simulink model "LATC_Test_Calc5000000"  (R2020b)
settings: Solver=FixedStepDiscrete  StartTime=4067.8601  StopTime=4107.8798  FixedStep=0.02  RelTol=1e-3
libraries: simulink x8
(part 2 of 2)

== matlab function LATC_Test_Calc5000000/MATLAB Function ==
  data: input input; y output; reset input; Tau input; b input; Ts input
function y = LatCtrlLeadFilter(input, reset, Tau, b, Ts)
%#codegen
%Description: Discrete implementation of the continious lead filter 
%G_lead_continious = (1+s*Tau)/(1+s*Tau) using Tustin transformation 
%(also known as bilinear transformation), hence s=2*(z-1)/(Ts*(z+1));

%--------------Inputs----------------------------------------------
%input                  input to lead filter
%reset                  Boolean indicating whether to reset the system
%Tau                    lead filter parameter, see Description section
%b                      Lead filter parameter, see Description section
% b=cot(Ts*wc/2)  双移线性变换 wc为截至频率
%Ts                     Sample time
%-------------------------------------------------------------------

%--------------Outputs----------------------------------------------
%y                     the output from the lead filter
%-------------------------------------------------------------------
persistent input_prev;
persistent output_prev;


if isempty(input_prev)
    input_prev = single(0);
end

if isempty(output_prev)
    output_prev = single(0);
end

if reset
    y = input;
else
    d1 = (b*Ts+2*Tau*b)/(b*Ts+2*Tau);
    d2 = (b*Ts-2*Tau*b)/(b*Ts+2*Tau);
    d3 = (b*Ts-2*Tau)/(b*Ts+2*Tau);
    y = input*d1+input_prev*d2-output_prev*d3; %compute output using tustin transformation
end

input_prev = input;
output_prev = y;

== matlab function LATC_Test_Calc5000000/MATLAB Function1 ==
  data: VxvRef input; AckConst output; Vch input; WheelBase input; AlpWheelAngle input; PsiDtAck output; Kap output
function [AckConst,PsiDtAck,Kap] = Ackman(VxvRef,Vch,WheelBase,AlpWheelAngle)
%#codegen
AckConst = single(zeros(1,1));
PsiDtAck = single(zeros(length(AlpWheelAngle),1));
Kap = single(zeros(length(AlpWheelAngle),1));
for i = 1:length(AlpWheelAngle)
    if VxvRef(i,1)==uint8(0)%转换常数数据类型
        PsiDtAck(i,1) = single(0);%转换常数数据类型
        AckConst = single(1);%转换常数数据类型
    else
        AckConst = min((single(1)+VxvRef(i,1)*VxvRef(i,1)/(Vch*Vch))*WheelBase/VxvRef(i,1),single(32767));%转换常数数据类型
        PsiDtAck(i,1) = AlpWheelAngle(i,1)/AckConst;
    end
    Kap(i,1) =  PsiDtAck(i,1)/max(VxvRef(i,1),0.5);
end
end

== matlab function LATC_Test_Calc5000000/MATLAB Function2 ==
  data: Delta_t input; tCycle input; dDeltaX output; KAP input; Vego input; dDeltaY output; CosOfPsi output; SinOfPsi output; t_Psi output
function [dDeltaX,dDeltaY,CosOfPsi,SinOfPsi,t_Psi] = EgoVehicleMovement(Delta_t,tCycle,KAP,Vego)
%#codegen
dDeltaX = single(0);
dDeltaY = single(0);
t_Psi = single(0);
CosOfPsi = single(0);
SinOfPsi = single(0);
KAP_Num = round(Delta_t/tCycle);
KAP_temp = KAP(length(KAP)-KAP_Num:1:end);
Vego = Vego(length(KAP)-KAP_Num:1:end);

for i = 1:length(KAP_temp)-1 % KAP 从最早时间开始排列
    Kap = KAP_temp(i);
    if Kap==0
        dDeltaX = dDeltaX + Vego(i)*tCycle;
        dDeltaY = dDeltaY + single(0);
        CosOfPsi = single(1);
        SinOfPsi = single(0);
    else
        d_Psi = Kap*Vego(i)*tCycle;
        SinOfPsi = sin(d_Psi);
        CosOfPsi = cos(d_Psi);
        dDeltaX = dDeltaX + SinOfPsi/Kap;
        dDeltaY = dDeltaY + 2*(sin(d_Psi/2)*sin(d_Psi/2))/Kap;
        t_Psi = t_Psi + d_Psi;
    end
end

== matlab function LATC_Test_Calc5000000/MATLAB Function4 ==
  data: Delta_t input; tCycle input; DeltaX output; KAP input; Vego input; DeltaY output; CosOfPsi output; SinOfPsi output; t_Psi output; LHA0 input; LHA1 input; LHA2 input; LHA3 input; LHC3 output; LHC2 output; LHC1 output; LHC0 output
function [DeltaX,DeltaY,CosOfPsi,SinOfPsi,t_Psi,LHC3,LHC2,LHC1,LHC0] = EgoVehicleMovement(Delta_t,tCycle,KAP,Vego,LHA0,LHA1,LHA2,LHA3)
%#codegen
% 线上取点
A = single(0);B = single(0);C = single(0);D = single(0);
temp_x = [0,20,40,80];
y1 = LHA0+LHA1*temp_x(1)+LHA2*temp_x(1)^2+LHA3*temp_x(1)^3;
y2 = LHA0+LHA1*temp_x(2)+LHA2*temp_x(2)^2+LHA3*temp_x(2)^3;
y3 = LHA0+LHA1*temp_x(3)+LHA2*temp_x(3)^2+LHA3*temp_x(3)^3;
y4 = LHA0+LHA1*temp_x(4)+LHA2*temp_x(4)^2+LHA3*temp_x(4)^3;
temp_y = [y1,y2,y3,y4];
%
DeltaX = single(0);
DeltaY = single(0);
t_Psi = single(0);
CosOfPsi = single(0);
SinOfPsi = single(0);

Step_Num = round(Delta_t/tCycle);
KAP_temp = KAP(length(KAP)-Step_Num:1:end);
Vego_temp = Vego(length(Vego)-Step_Num:1:end);

for i = 1:length(KAP_temp)-1 % KAP 从最早时间开始排列
    Kap = KAP_temp(i);
    if Kap==0
        d_Psi = single(0);
        CosOfPsi = single(1);
        SinOfPsi = single(0);
        dDeltaX = Vego_temp(i)*tCycle;
        dDeltaY = single(0);
        
        t_Psi = t_Psi + d_Psi;
        DeltaX = DeltaX + dDeltaX;
        DeltaY = DeltaY + dDeltaY;

    else
        d_Psi = Kap*Vego_temp(i)*tCycle;
        SinOfPsi = sin(d_Psi);
        CosOfPsi = cos(d_Psi);
        dDeltaX = SinOfPsi/Kap;
        dDeltaY = 2*(sin(d_Psi/2)*sin(d_Psi/2))/Kap;

        t_Psi = t_Psi + d_Psi;
        DeltaX = DeltaX + dDeltaX;
        DeltaY = DeltaY + dDeltaY;
    end
    t_dx = temp_x-dDeltaX;
    t_dy = temp_y-dDeltaY;
    Temp_X = t_dx*CosOfPsi+t_dy*SinOfPsi;
    Temp_Y = -t_dx*SinOfPsi+t_dy*CosOfPsi;
    [A,B,C,D] = pl(Temp_X,Temp_Y);
    temp_x = [0,20,40,80];
    y1 = D+C*temp_x(1)+B*temp_x(1)^2+A*temp_x(1)^3;
    y2 = D+C*temp_x(2)+B*temp_x(2)^2+A*temp_x(2)^3;
    y3 = D+C*temp_x(3)+B*temp_x(3)^2+A*temp_x(3)^3;
    y4 = D+C*temp_x(4)+B*temp_x(4)^2+A*temp_x(4)^3;
    temp_y = [y1,y2,y3,y4];
end
LHC3 = A;
LHC2 = B;
LHC1 = C;
LHC0 = D;
end
 function [A,B,C,D] = pl(X,Y)
MatrixA = [X(1)^3,X(1)^2,X(1),1;...
           X(2)^3,X(2)^2,X(2),1;...
           X(3)^3,X(3)^2,X(3),1;...
           X(4)^3,X(4)^2,X(4),1];
MatrixB = [Y(1);Y(2);Y(3);Y(4)];
if det(MatrixA)==0
    A=cast(0,class(X(1)));
    B=cast(0,class(X(1)));
    C=cast(0,class(X(1)));
    D=cast(0,class(X(1)));
else
    P = MatrixA\MatrixB;
    A = P(1);
    B = P(2);
    C = P(3);
    D = P(4);
end
% coder.allowpcode('plain');
end

== matlab function LATC_Test_Calc5000000/MATLAB Function5 ==
  data: dDeltaX input; LHC3 output; dDeltaY input; CosOfPsi input; SinOfPsi input; LHA0 input; LHA1 input; LHA2 input; LHA3 input; range input; LHC2 output; LHC1 output; LHC0 output
function [LHC3,LHC2,LHC1,LHC0] = fcn(dDeltaX,dDeltaY,CosOfPsi,SinOfPsi,LHA0,LHA1,LHA2,LHA3,range)

 % temp_x = [0,1/4*range,1/2*range,range];
 temp_x = [0,20,40,80];
  
 y1 = LHA0+LHA1*temp_x(1)+LHA2*temp_x(1)^2+LHA3*temp_x(1)^3;
 y2 = LHA0+LHA1*temp_x(2)+LHA2*temp_x(2)^2+LHA3*temp_x(2)^3;
 y3 = LHA0+LHA1*temp_x(3)+LHA2*temp_x(3)^2+LHA3*temp_x(3)^3;
 y4 = LHA0+LHA1*temp_x(4)+LHA2*temp_x(4)^2+LHA3*temp_x(4)^3;
 temp_y = [y1,y2,y3,y4];
 t_dx = temp_x-dDeltaX;
 t_dy = temp_y-dDeltaY;
 TmpX = t_dx*CosOfPsi+t_dy*SinOfPsi;
 TmpY = -t_dx*SinOfPsi+t_dy*CosOfPsi;
%  P = polyfit(TmpX,TmpY,3);
%  LHC3 = P(1);
%  LHC2 = P(2);
%  LHC1 = P(3);
%  LHC0 = P(4);
 [A,B,C,D] = pl(TmpX,TmpY);
 LHC3 = A;
 LHC2 = B;
 LHC1 = C;
 LHC0 = D;
end
 function [A,B,C,D] = pl(X,Y)
MatrixA = [X(1)^3,X(1)^2,X(1),1;...
           X(2)^3,X(2)^2,X(2),1;...
           X(3)^3,X(3)^2,X(3),1;...
           X(4)^3,X(4)^2,X(4),1];
MatrixB = [Y(1);Y(2);Y(3);Y(4)];
if det(MatrixA)==0
    A=cast(0,class(X(1)));
    B=cast(0,class(X(1)));
    C=cast(0,class(X(1)));
    D=cast(0,class(X(1)));
else
    P = MatrixA\MatrixB;
    A = P(1);
    B = P(2);
    C = P(3);
    D = P(4);
end
% coder.allowpcode('plain');
end
